simulink model "CTRL_SPECCTRL_FF_ACCPED_test"  (R2024b)
settings: Solver=VariableStepAuto  StartTime=0.0  StopTime=10.0  RelTol=1e-3
libraries: CTRL_SPECCTRL_FF_ACCPED x1
settings Model: Creator=blatak  LastModifiedBy=blatak

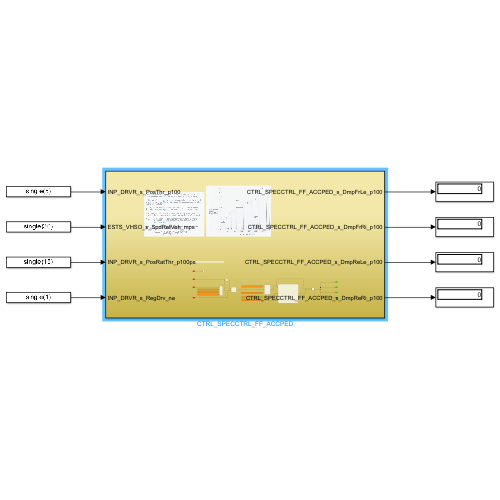
[thumbnail: Simulink's stored preview of the top-level diagram]
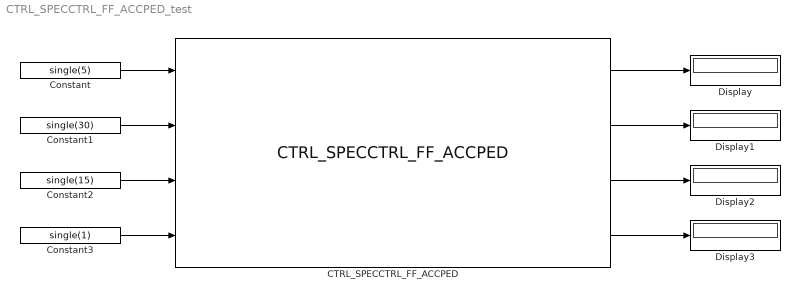
== system CTRL_SPECCTRL_FF_ACCPED_test ==
  CTRL_SPECCTRL_FF_ACCPED : CTRL_SPECCTRL_FF_ACCPED/CTRL_SPECCTRL_FF_ACCPED  SystemSampleTime=-1  VariantActivationTime=update diagram  AllowFlexibleInterface=on  Latency=0  AutoFrameSizeCalculation=off
  Constant : Constant  Value=single(5)
  Constant1 : Constant  Value=single(30)
  Constant2 : Constant  Value=single(15)
  Constant3 : Constant  Value=single(1)
  Display{,1..3} (4 alike) : Display
  wires:
  CTRL_SPECCTRL_FF_ACCPED/1 -> Display/1
  CTRL_SPECCTRL_FF_ACCPED/2 -> Display1/1
  CTRL_SPECCTRL_FF_ACCPED/3 -> Display2/1
  CTRL_SPECCTRL_FF_ACCPED/4 -> Display3/1
  Constant/1 -> CTRL_SPECCTRL_FF_ACCPED/1
  Constant1/1 -> CTRL_SPECCTRL_FF_ACCPED/2
  Constant2/1 -> CTRL_SPECCTRL_FF_ACCPED/3
  Constant3/1 -> CTRL_SPECCTRL_FF_ACCPED/4
